simulink model "VECTOR_CONTROL_FOC_OF_IM_2023"  (R2023b)
settings: Solver=FixedStepDiscrete  StartTime=0.0  StopTime=1  RelTol=1e-3
PreLoadFcn:
  | Ts=2e-6;
InitFcn:
  | clc;
  | clear all;
  | % All Parameters
  | Ts=2e-6; %Sampling time
  | S=50*746; %nominal power
  | Vs=460; %Stator voltage
  | f=50; %Supply frequency
  | Rs=0.087; %Stator resistance
  | Rr=0.228; %Rotor resistance
  | Lls=0.0001; %Stator inductance
  | Llr=0.0008; %Rotor inductance
  | Lm=0.0347;
  | P=4; %Number of Poles
  | Tr=(Llr+Lm)/Rr; %Time constant
  | J=0.662; %Inertia
  | F=0.1; %Friction factor
  | Ls=Lls+Lm;
  | Lr=Llr+Lm;
undefined symbols (not defined in the file): DiscIntNeverNeededParam
libraries: slpidlib x3, spsVoltageMeasurementLib x3, spsAsynchronousMachineSIUnitsLib x1, spsSawtoothGeneratorLib x1, simulink_extras x1, spsUniversalBridgeLib x1, spsDCVoltageSourceLib x1, sps_lib x1, spsStairGeneratorLib x1
settings Model: Creator=ShahRukh
settings SolverCC: AlgebraicLoopSolver=TrustRegion
settings DataIOCC: ReturnWorkspaceOutputs=off
settings DebuggingCC: UnconnectedInputMsg=warning  UnconnectedOutputMsg=warning  UnconnectedLineMsg=warning  ArithmeticOperatorsInVariantConditions=warning
settings ModelReferenceCC: EnableRefExpFcnMdlSchedulingChecks=on
settings SFSimCC: SimUseLocalCustomCode=off  CustomCodeUndefinedFunction=UseInterfaceOnly
settings RTWCC: RTWUseLocalCustomCode=off
settings ConfigComp: CovBoundaryAbsTol=1.0e-5
settings SimscapeCC: SimscapeLogDataHistory=10000

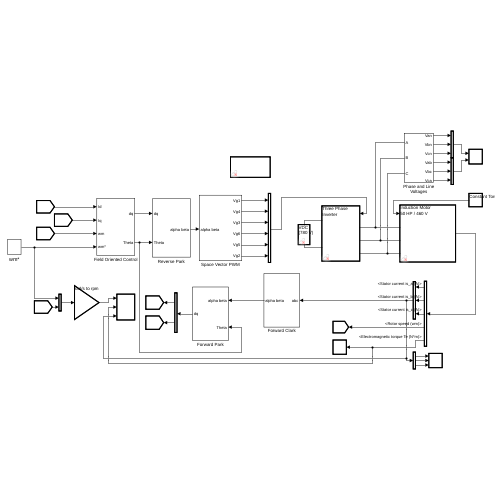
[thumbnail: Simulink's stored preview of the top-level diagram]
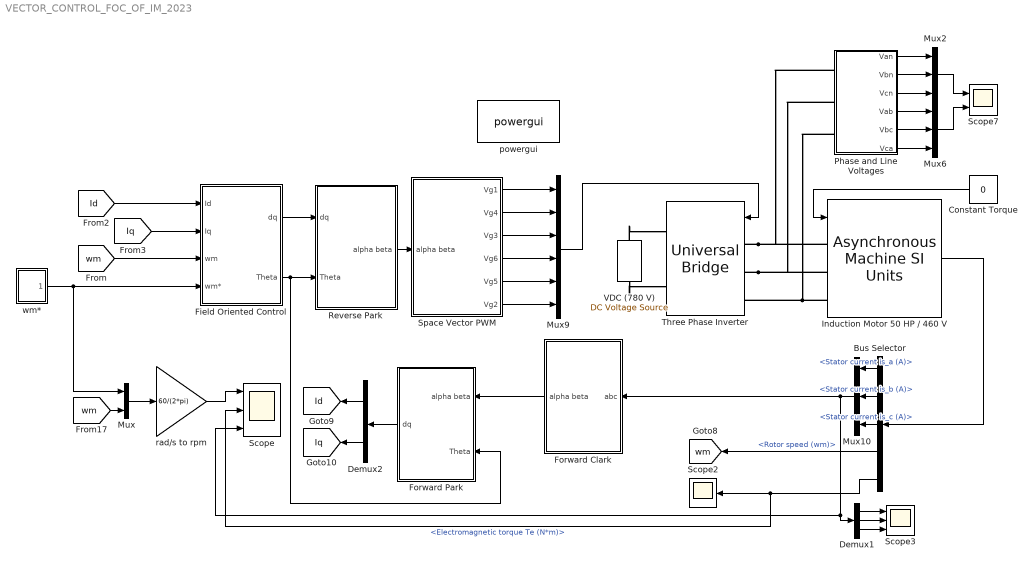
== system VECTOR_CONTROL_FOC_OF_IM_2023 ==
  Bus Selector : BusSelector  OutputSignals=Stator measurements.Stator current is_a (A),Stator measurements.Stator current is_b (A),Stator measurements.Stator current is_c (A),Mechanical.Rotor speed (wm),Mechanical.Electromagnetic torque Te (N*m)
  Constant Torque : Constant  Value=0
  Demux1 : Demux  Outputs=3
  Demux2 : Demux  Outputs=2
  Field Oriented Control : Subsystem
  Forward Clark : Subsystem
  Forward Park : Subsystem
  Induction Motor 50 HP / 460 V : spsAsynchronousMachineSIUnitsLib/Asynchronous Machine SI Units  RotorType=Squirrel-cage  PresetModel=No  MechanicalLoad=Torque Tm  ShowDetailedParameters=on  ReferenceFrame=Stationary  Units=SI  MeasurementBus=off  NominalParameters=[ S, Vs, f ]  VoltageRatio=1  Stator=[ Rs Lls ]  Rotor="[ Rr  Llr ]"  Cage1=[ 0.022 0.226/377]  Cage2=[ 0.022 0.226/377]  Lm=Lm  Mechanical="[J  F P/2 ]"  PolePairs=2  InitialConditions="[ 1, 0 ,  0 , 0 , 0 , 0 , 0 , 0 ]"  SimulateSaturation=off  Saturation=[0 0;0 0]  LoadFlowParameters=0  TsPowergui=0  TsBlock=-1  IterativeModel=Trapezoidal non iterative  IterativeDiscreteModel=Trapezoidal non iterative  Pmec=0
      settings: AttributesFormatString=\n
  Mux : Mux  Inputs=2
  Mux10 : Mux  Inputs=3
  Mux2 : Mux  Inputs=3
  Mux6 : Mux  Inputs=3
  Mux9 : Mux  Inputs=6
  Phase and Line Voltages : Subsystem
  Reverse Park : Subsystem
  Scope : Scope  NumInputPorts=3
  Scope2 : Scope
  Scope3 : Scope  NumInputPorts=3
  Scope7 : Scope  NumInputPorts=2
  Space Vector PWM : Subsystem
  Three Phase Inverter : spsUniversalBridgeLib/Universal Bridge  Arms=3  SnubberResistance=1000  SnubberCapacitance=inf  Device=IGBT / Diodes  Ron=1e-3  Lon=0  ForwardVoltages="[  0.8  0.8  ]"  ForwardVoltage=.8  GTOparameters=[ 1e-6 , 1e-6 ]  IGBTparameters=[ 1e-6 , 2e-6 ]  Measurements=None  Measurements_2=None  converterType=Rectifier
      settings: AttributesFormatString=\n
  VDC (780 V) : spsDCVoltageSourceLib/DC Voltage Source  Description=source block  Amplitude=780  Measurements=None
      settings: AttributesFormatString=\n
  powergui : sps_lib/powergui  Priority=2  SimulationMode=Discrete  SampleTime=Ts  frequency=60  Iterations=50  frequencyindice=0  Pbase=100e6  ErrMax=1e-4  UnitsV=kV  UnitsW=MW  buscounter=0  FunctionMessages=off  echomessages=off  EnableUseOfTLC=off  CurrentSourceSwitches=off  DisableSnubberDevices=off  DisableRonSwitches=off  DisableVfSwitches=off  DisplayEquations=off  AutomaticDiscreteSolvers=off  SolverType=Tustin  Interpol=off  ExternalGateDelay=off  methode=off  Ts=0  x0status=blocks  SPID=off  SwTol=0  HookPort=off  NonlinearTolerance=1e-4  nMaxIteration=100  ContinueOnMaxIteration=off  RestoreLinks=warning  ResistiveCurrentMeasurement=off  Frange=[0:2:500]  Ylog=off  Xlog=on  ShowGrid=off  save=off  variable=ZData  structure=0  ZoomFFT=on  StartTime=0.0  cycles=1  DisplayStyle=off  fundamental=60  FreqAxis=off  MaxFrequency=1000  frequencyindicesteady=1  RmsSteady=1  display=off
  rad/s to rpm : Gain  Gain=60/(2*pi)
  wm* : Subsystem
  tag scope: Id=global, Iq=global, wm=global
  wires:
  Bus Selector/4 -> [wm]  "<Rotor speed (wm)>"
  Mux10/1 -> Scope/3, Demux1/1, Forward Clark/1(abc)
  Demux2/1 -> [Id]
  Mux6/1 -> Scope7/2
  Space Vector PWM/6(Vg2) -> Mux9/6
  Constant Torque/1 -> Induction Motor 50 HP / 460 V/1
  Phase and Line Voltages/3(Vcn) -> Mux2/3
  Phase and Line Voltages/5(Vbc) -> Mux6/2
  Space Vector PWM/2(Vg4) -> Mux9/2
  Phase and Line Voltages/2(Vbn) -> Mux2/2
  Mux2/1 -> Scope7/1
  Space Vector PWM/5(Vg5) -> Mux9/5
  Phase and Line Voltages/1(Van) -> Mux2/1
  Phase and Line Voltages/6(Vca) -> Mux6/3
  Bus Selector/2 -> Mux10/2  "<Stator current is_b (A)>"
  Forward Park/1(dq) -> Demux2/1
  Demux2/2 -> [Iq]
  Bus Selector/5 -> Scope/2, Scope2/1  "<Electromagnetic torque Te (N*m)>"
  Mux9/1 -> Three Phase Inverter/1
  Bus Selector/1 -> Mux10/1  "<Stator current is_a (A)>"
  Forward Clark/1(alpha beta) -> Forward Park/1(alpha beta)
  Phase and Line Voltages/4(Vab) -> Mux6/1
  Mux/1 -> rad/s to rpm/1
  Space Vector PWM/3(Vg3) -> Mux9/3
  [wm] -> Mux/2
  Induction Motor 50 HP / 460 V/1 -> Bus Selector/1
  Space Vector PWM/1(Vg1) -> Mux9/1
  rad/s to rpm/1 -> Scope/1
  Space Vector PWM/4(Vg6) -> Mux9/4
  Reverse Park/1(alpha beta) -> Space Vector PWM/1(alpha beta)
  Field Oriented Control/1(dq) -> Reverse Park/1(dq)
  Bus Selector/3 -> Mux10/3  "<Stator current is_c (A)>"
  wm*/1(" ") -> Mux/1, Field Oriented Control/4(wm*)
  [wm] -> Field Oriented Control/3(wm)
  [Id] -> Field Oriented Control/1(Id)
  [Iq] -> Field Oriented Control/2(Iq)
  Field Oriented Control/2(Theta) -> Forward Park/2(Theta), Reverse Park/2(Theta)
  Demux1/1 -> Scope3/1
  Demux1/2 -> Scope3/2
  Demux1/3 -> Scope3/3
  connections:
  Three Phase Inverter/LConn1 -- Induction Motor 50 HP / 460 V/LConn1 -- Phase and Line Voltages/LConn1
  Induction Motor 50 HP / 460 V/LConn3 -- Three Phase Inverter/LConn3 -- Phase and Line Voltages/LConn3
  Three Phase Inverter/LConn2 -- Induction Motor 50 HP / 460 V/LConn2 -- Phase and Line Voltages/LConn2
  VDC (780 V)/RConn1 -- Three Phase Inverter/RConn1
  VDC (780 V)/LConn1 -- Three Phase Inverter/RConn2

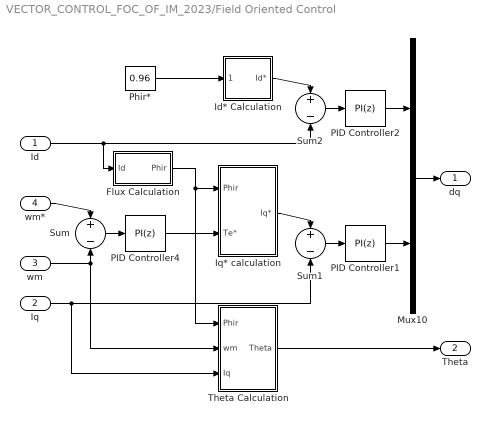
== system VECTOR_CONTROL_FOC_OF_IM_2023/Field Oriented Control ==
  Id : Inport
  Iq : Inport  Port=2
  wm : Inport  Port=3
  wm* : Inport  Port=4
  Flux Calculation : Subsystem  mask(Flux Calcultation){}
      mask init:
      | NF=0.44572610323020e-6;
      | DF=[1 -0.99998715486734];
  Id* Calculation : Subsystem
  Iq* calculation : Subsystem
  Mux10 : Mux  Inputs=2
  PID Controller1 : slpidlib/PID Controller  Controller=PI  Form=Parallel  TimeDomain=Discrete-time  UseExternalTs=off  SampleTime=-1  IntegratorMethod=Forward Euler  FilterMethod=Forward Euler  ControllerParametersSource=internal  P=100  I=26  UseKiTs=off  D=30  N=100  UseFilter=on  TunerSelectOption=Transfer Function Based (PID Tuner App)  InitialConditionSource=internal  InitialConditionForIntegrator=0  InitialConditionForFilter=0  DifferentiatorICPrevScaledInput=0  ExternalReset=none  TrackingMode=off  Kt=1  LimitOutput=off  SatLimitsSource=internal  UpperSaturationLimit=inf  LowerSaturationLimit=-inf  LinearizeAsGain=on  AntiWindupMode=none  Kb=1  LimitIntegrator=off  UpperIntegratorSaturationLimit=inf  LowerIntegratorSaturationLimit=-inf  POutMin=[]  POutMax=[]  IOutMin=[]  IOutMax=[]  DOutMin=[]  DOutMax=[]  NOutMin=[]  NOutMax=[]  SumOutMin=[]  SumOutMax=[]  SaturationOutMin=[]  SaturationOutMax=[]  PParamMin=[]  PParamMax=[]  IParamMin=[]  IParamMax=[]  DParamMin=[]  DParamMax=[]  NParamMin=[]  NParamMax=[]  KbParamMin=[]  KbParamMax=[]  KtParamMin=[]  KtParamMax=[]  KbOutMin=[]  KbOutMax=[]  KtOutMin=[]  KtOutMax=[]  IntegratorOutMin=[]  IntegratorOutMax=[]  FilterOutMin=[]  FilterOutMax=[]  SumI1OutMin=[]  SumI1OutMax=[]  SumI2OutMin=[]  SumI2OutMax=[]  SumI3OutMin=[]  SumI3OutMax=[]  SumI4OutMin=[]  SumI4OutMax=[]  SumDOutMin=[]  SumDOutMax=[]  DifferentiatorOutMin=[]  DifferentiatorOutMax=[]  FilterDiffOutCoefMin=[]  FilterDiffOutCoefMax=[]  ReciprocalOutMin=[]  ReciprocalOutMax=[]  SumDenOutMin=[]  SumDenOutMax=[]  SumNumOutMin=[]  SumNumOutMax=[]  DivideOutMin=[]  DivideOutMax=[]  UdiffTsProdOutMin=[]  UdiffTsProdOutMax=[]  NTsProdOutMin=[]  NTsProdOutMax=[]  UintegralTsProdOutMin=[]  UintegralTsProdOutMax=[]  UngainTsProdOutMin=[]  UngainTsProdOutMax=[]  ClampingZeroOutDataTypeStr=Inherit: Inherit via back propagation  ClampingZeroOutMin=[]  ClampingZeroOutMax=[]  FilterDenConstantOutDataTypeStr=Inherit: Inherit via back propagation  FilterDenConstantOutMin=[]  FilterDenConstantOutMax=[]  PCopyOutDataTypeStr=Inherit: Inherit via back propagation  PCopyOutMin=[]  PCopyOutMax=[]  NCopyOutDataTypeStr=Inherit: Inherit via back propagation  NCopyOutMin=[]  NCopyOutMax=[]  IntegratorContinuousStateAttributes=''  IntegratorStateMustResolveToSignalObject=off  IntegratorRTWStateStorageClass=Auto  FilterContinuousStateAttributes=''  FilterStateMustResolveToSignalObject=off  FilterRTWStateStorageClass=Auto  ParallelPVariant=InternalParameters  IdealPVariant=Disabled  IVariant=InternalParameters  DVariant=Disabled  IntegratorVariant=Discrete  SatVariant=Disabled  AWVariant=Passthrough  PCopyVariant=Disabled  TRVariant=Disabled  FdbkBlocksVariant=Forward  IdealPFdbkVariant=Disabled  SatFdbkVariant=Disabled  DerivativeFilterVariant=Disabled  NVariant=Disabled  NCopyVariant=Disabled_SignalSpec  FilterICVariant=Disabled  IntegratorICVariant=InternalICs  ExternalResetVariant=Disabled  TRSumVariant=Passthrough  SumFdbkVariant=Disabled  SumVariant=Sum_PI  TsampFilterVariant=InternalTs  TsampNgainVariant=Passthrough  TsampIntegralVariant=Disabled_SignalSpec  ExternalSaturationOutDataTypeStr=Inherit: Same as second input
  PID Controller2 : slpidlib/PID Controller  Controller=PI  Form=Parallel  TimeDomain=Discrete-time  UseExternalTs=off  SampleTime=-1  IntegratorMethod=Forward Euler  FilterMethod=Forward Euler  ControllerParametersSource=internal  P=100  I=26  UseKiTs=off  D=30  N=100  UseFilter=on  TunerSelectOption=Transfer Function Based (PID Tuner App)  InitialConditionSource=internal  InitialConditionForIntegrator=0  InitialConditionForFilter=0  DifferentiatorICPrevScaledInput=0  ExternalReset=none  TrackingMode=off  Kt=1  LimitOutput=off  SatLimitsSource=internal  UpperSaturationLimit=inf  LowerSaturationLimit=-inf  LinearizeAsGain=on  AntiWindupMode=none  Kb=1  LimitIntegrator=off  UpperIntegratorSaturationLimit=inf  LowerIntegratorSaturationLimit=-inf  POutMin=[]  POutMax=[]  IOutMin=[]  IOutMax=[]  DOutMin=[]  DOutMax=[]  NOutMin=[]  NOutMax=[]  SumOutMin=[]  SumOutMax=[]  SaturationOutMin=[]  SaturationOutMax=[]  PParamMin=[]  PParamMax=[]  IParamMin=[]  IParamMax=[]  DParamMin=[]  DParamMax=[]  NParamMin=[]  NParamMax=[]  KbParamMin=[]  KbParamMax=[]  KtParamMin=[]  KtParamMax=[]  KbOutMin=[]  KbOutMax=[]  KtOutMin=[]  KtOutMax=[]  IntegratorOutMin=[]  IntegratorOutMax=[]  FilterOutMin=[]  FilterOutMax=[]  SumI1OutMin=[]  SumI1OutMax=[]  SumI2OutMin=[]  SumI2OutMax=[]  SumI3OutMin=[]  SumI3OutMax=[]  SumI4OutMin=[]  SumI4OutMax=[]  SumDOutMin=[]  SumDOutMax=[]  DifferentiatorOutMin=[]  DifferentiatorOutMax=[]  FilterDiffOutCoefMin=[]  FilterDiffOutCoefMax=[]  ReciprocalOutMin=[]  ReciprocalOutMax=[]  SumDenOutMin=[]  SumDenOutMax=[]  SumNumOutMin=[]  SumNumOutMax=[]  DivideOutMin=[]  DivideOutMax=[]  UdiffTsProdOutMin=[]  UdiffTsProdOutMax=[]  NTsProdOutMin=[]  NTsProdOutMax=[]  UintegralTsProdOutMin=[]  UintegralTsProdOutMax=[]  UngainTsProdOutMin=[]  UngainTsProdOutMax=[]  ClampingZeroOutDataTypeStr=Inherit: Inherit via back propagation  ClampingZeroOutMin=[]  ClampingZeroOutMax=[]  FilterDenConstantOutDataTypeStr=Inherit: Inherit via back propagation  FilterDenConstantOutMin=[]  FilterDenConstantOutMax=[]  PCopyOutDataTypeStr=Inherit: Inherit via back propagation  PCopyOutMin=[]  PCopyOutMax=[]  NCopyOutDataTypeStr=Inherit: Inherit via back propagation  NCopyOutMin=[]  NCopyOutMax=[]  IntegratorContinuousStateAttributes=''  IntegratorStateMustResolveToSignalObject=off  IntegratorRTWStateStorageClass=Auto  FilterContinuousStateAttributes=''  FilterStateMustResolveToSignalObject=off  FilterRTWStateStorageClass=Auto  ParallelPVariant=InternalParameters  IdealPVariant=Disabled  IVariant=InternalParameters  DVariant=Disabled  IntegratorVariant=Discrete  SatVariant=Disabled  AWVariant=Passthrough  PCopyVariant=Disabled  TRVariant=Disabled  FdbkBlocksVariant=Forward  IdealPFdbkVariant=Disabled  SatFdbkVariant=Disabled  DerivativeFilterVariant=Disabled  NVariant=Disabled  NCopyVariant=Disabled_SignalSpec  FilterICVariant=Disabled  IntegratorICVariant=InternalICs  ExternalResetVariant=Disabled  TRSumVariant=Passthrough  SumFdbkVariant=Disabled  SumVariant=Sum_PI  TsampFilterVariant=InternalTs  TsampNgainVariant=Passthrough  TsampIntegralVariant=Disabled_SignalSpec  ExternalSaturationOutDataTypeStr=Inherit: Same as second input
  PID Controller4 : slpidlib/PID Controller  Controller=PI  Form=Parallel  TimeDomain=Discrete-time  UseExternalTs=off  SampleTime=-1  IntegratorMethod=Forward Euler  FilterMethod=Forward Euler  ControllerParametersSource=internal  P=20  I=26  UseKiTs=off  D=0  N=100  UseFilter=on  TunerSelectOption=Transfer Function Based (PID Tuner App)  InitialConditionSource=internal  InitialConditionForIntegrator=0  InitialConditionForFilter=0  DifferentiatorICPrevScaledInput=0  ExternalReset=none  TrackingMode=off  Kt=1  LimitOutput=off  SatLimitsSource=internal  UpperSaturationLimit=600  LowerSaturationLimit=-600  LinearizeAsGain=on  AntiWindupMode=none  Kb=1  LimitIntegrator=off  UpperIntegratorSaturationLimit=inf  LowerIntegratorSaturationLimit=-inf  POutMin=[]  POutMax=[]  IOutMin=[]  IOutMax=[]  DOutMin=[]  DOutMax=[]  NOutMin=[]  NOutMax=[]  SumOutMin=[]  SumOutMax=[]  SaturationOutMin=[]  SaturationOutMax=[]  PParamMin=[]  PParamMax=[]  IParamMin=[]  IParamMax=[]  DParamMin=[]  DParamMax=[]  NParamMin=[]  NParamMax=[]  KbParamMin=[]  KbParamMax=[]  KtParamMin=[]  KtParamMax=[]  KbOutMin=[]  KbOutMax=[]  KtOutMin=[]  KtOutMax=[]  IntegratorOutMin=[]  IntegratorOutMax=[]  FilterOutMin=[]  FilterOutMax=[]  SumI1OutMin=[]  SumI1OutMax=[]  SumI2OutMin=[]  SumI2OutMax=[]  SumI3OutMin=[]  SumI3OutMax=[]  SumI4OutMin=[]  SumI4OutMax=[]  SumDOutMin=[]  SumDOutMax=[]  DifferentiatorOutMin=[]  DifferentiatorOutMax=[]  FilterDiffOutCoefMin=[]  FilterDiffOutCoefMax=[]  ReciprocalOutMin=[]  ReciprocalOutMax=[]  SumDenOutMin=[]  SumDenOutMax=[]  SumNumOutMin=[]  SumNumOutMax=[]  DivideOutMin=[]  DivideOutMax=[]  UdiffTsProdOutMin=[]  UdiffTsProdOutMax=[]  NTsProdOutMin=[]  NTsProdOutMax=[]  UintegralTsProdOutMin=[]  UintegralTsProdOutMax=[]  UngainTsProdOutMin=[]  UngainTsProdOutMax=[]  ClampingZeroOutDataTypeStr=Inherit: Inherit via back propagation  ClampingZeroOutMin=[]  ClampingZeroOutMax=[]  FilterDenConstantOutDataTypeStr=Inherit: Inherit via back propagation  FilterDenConstantOutMin=[]  FilterDenConstantOutMax=[]  PCopyOutDataTypeStr=Inherit: Inherit via back propagation  PCopyOutMin=[]  PCopyOutMax=[]  NCopyOutDataTypeStr=Inherit: Inherit via back propagation  NCopyOutMin=[]  NCopyOutMax=[]  IntegratorContinuousStateAttributes=''  IntegratorStateMustResolveToSignalObject=off  IntegratorRTWStateStorageClass=Auto  FilterContinuousStateAttributes=''  FilterStateMustResolveToSignalObject=off  FilterRTWStateStorageClass=Auto  ParallelPVariant=InternalParameters  IdealPVariant=Disabled  IVariant=InternalParameters  DVariant=Disabled  IntegratorVariant=Discrete  SatVariant=Disabled  AWVariant=Passthrough  PCopyVariant=Disabled  TRVariant=Disabled  FdbkBlocksVariant=Forward  IdealPFdbkVariant=Disabled  SatFdbkVariant=Disabled  DerivativeFilterVariant=Disabled  NVariant=Disabled  NCopyVariant=Disabled_SignalSpec  FilterICVariant=Disabled  IntegratorICVariant=InternalICs  ExternalResetVariant=Disabled  TRSumVariant=Passthrough  SumFdbkVariant=Disabled  SumVariant=Sum_PI  TsampFilterVariant=InternalTs  TsampNgainVariant=Passthrough  TsampIntegralVariant=Disabled_SignalSpec  ExternalSaturationOutDataTypeStr=Inherit: Same as second input
  Phir* : Constant  Value=0.96
  Sum : Sum  Inputs=+-
  Sum1 : Sum  Inputs=+-
  Sum2 : Sum  Inputs=+-
  Theta Calculation : Subsystem
  dq : Outport  VectorParamsAs1DForOutWhenUnconnected=off
  Theta : Outport  Port=2  VectorParamsAs1DForOutWhenUnconnected=off
  wires:
  wm*/1 -> Sum/1
  Phir*/1 -> Id* Calculation/1(Phir*)
  Iq* calculation/1(Iq*) -> Sum1/1
  wm/1 -> Theta Calculation/2(wm), Sum/2
  Theta Calculation/1(Theta) -> Theta/1
  Id/1 -> Flux Calculation/1(Id), Sum2/2
  Mux10/1 -> dq/1
  Id* Calculation/1(Id*) -> Sum2/1
  PID Controller4/1 -> Iq* calculation/2(Te*)
  Sum1/1 -> PID Controller1/1
  Iq/1 -> Sum1/2, Theta Calculation/3(Iq)
  PID Controller2/1 -> Mux10/1
  PID Controller1/1 -> Mux10/2
  Sum2/1 -> PID Controller2/1
  Sum/1 -> PID Controller4/1
  Flux Calculation/1(Phir) -> Theta Calculation/1(Phir), Iq* calculation/1(Phir)

== system VECTOR_CONTROL_FOC_OF_IM_2023/Forward Clark ==
  abc : Inport
  Mux5 : Mux  Inputs=2
  alpha : Fcn  Expr=((2/3)*u(1))-((1/3)*u(2))-((1/3)*u(3))
  beta : Fcn  Expr=((0)*u(1))+((1/sqrt(3))*u(2))-((1/sqrt(3))*u(3))
  alpha beta : Outport  VectorParamsAs1DForOutWhenUnconnected=off
  wires:
  Mux5/1 -> alpha beta/1
  alpha/1 -> Mux5/1
  beta/1 -> Mux5/2
  abc/1 -> beta/1, alpha/1

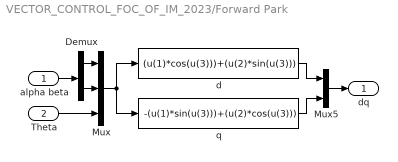
== system VECTOR_CONTROL_FOC_OF_IM_2023/Forward Park ==
  alpha beta : Inport
  Theta : Inport  Port=2
  Demux : Demux  Outputs=2
  Mux : Mux  Inputs=3
  Mux5 : Mux  Inputs=2
  d : Fcn  Expr=(u(1)*cos(u(3)))+(u(2)*sin(u(3)))
  q : Fcn  Expr=-(u(1)*sin(u(3)))+(u(2)*cos(u(3)))
  dq : Outport  VectorParamsAs1DForOutWhenUnconnected=off
  wires:
  Mux5/1 -> dq/1
  d/1 -> Mux5/1
  q/1 -> Mux5/2
  Mux/1 -> q/1, d/1
  alpha beta/1 -> Demux/1
  Demux/1 -> Mux/1
  Demux/2 -> Mux/2
  Theta/1 -> Mux/3

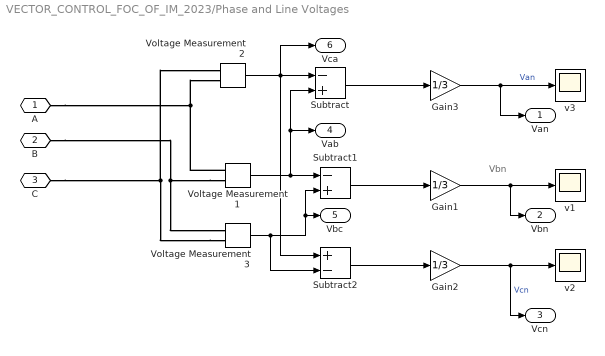
== system VECTOR_CONTROL_FOC_OF_IM_2023/Phase and Line Voltages ==
  note: Vbn
  Gain1 : Gain  Gain=1/3
  Gain2 : Gain  Gain=1/3
  Gain3 : Gain  Gain=1/3
  Subtract : Sum  Inputs=-+
  Subtract1 : Sum  Inputs=-+
  Subtract2 : Sum  Inputs=+-
  Voltage Measurement1 : spsVoltageMeasurementLib/Voltage Measurement  PhasorSimulation=off  OutputType=Complex  PSBequivalent=0
  Voltage Measurement2 : spsVoltageMeasurementLib/Voltage Measurement  PhasorSimulation=off  OutputType=Complex  PSBequivalent=0
  Voltage Measurement3 : spsVoltageMeasurementLib/Voltage Measurement  PhasorSimulation=off  OutputType=Complex  PSBequivalent=0
  v1 : Scope
  v2 : Scope
  v3 : Scope
  A : PMIOPort  Side=Left
  B : PMIOPort  Port=2  Side=Left
  C : PMIOPort  Port=3  Side=Left
  Van : Outport  VectorParamsAs1DForOutWhenUnconnected=off
  Vbn : Outport  Port=2  VectorParamsAs1DForOutWhenUnconnected=off
  Vcn : Outport  Port=3  VectorParamsAs1DForOutWhenUnconnected=off
  Vab : Outport  Port=4  VectorParamsAs1DForOutWhenUnconnected=off
  Vbc : Outport  Port=5  VectorParamsAs1DForOutWhenUnconnected=off
  Vca : Outport  Port=6  VectorParamsAs1DForOutWhenUnconnected=off
  wires:
  Gain2/1 -> v2/1, Vcn/1  "Vcn"
  Subtract2/1 -> Gain2/1
  Gain1/1 -> v1/1, Vbn/1
  Subtract1/1 -> Gain1/1
  Voltage Measurement3/1 -> Subtract1/2, Vbc/1, Subtract2/2
  Gain3/1 -> v3/1, Van/1  "Van"
  Subtract/1 -> Gain3/1
  Voltage Measurement1/1 -> Vab/1, Subtract/2, Subtract1/1
  Voltage Measurement2/1 -> Vca/1, Subtract2/1, Subtract/1
  connections:
  Voltage Measurement1/LConn1 -- A/RConn1 -- Voltage Measurement2/LConn2
  Voltage Measurement1/LConn2 -- B/RConn1 -- Voltage Measurement3/LConn1
  Voltage Measurement3/LConn2 -- Voltage Measurement2/LConn1 -- C/RConn1

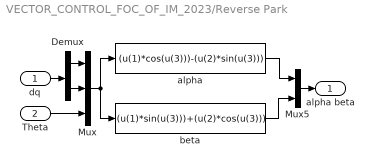
== system VECTOR_CONTROL_FOC_OF_IM_2023/Reverse Park ==
  dq : Inport
  Theta : Inport  Port=2
  Demux : Demux  Outputs=2
  Mux : Mux  Inputs=3
  Mux5 : Mux  Inputs=2
  alpha : Fcn  Expr=(u(1)*cos(u(3)))-(u(2)*sin(u(3)))
  beta : Fcn  Expr=(u(1)*sin(u(3)))+(u(2)*cos(u(3)))
  alpha beta : Outport  VectorParamsAs1DForOutWhenUnconnected=off
  wires:
  Mux5/1 -> alpha beta/1
  alpha/1 -> Mux5/1
  beta/1 -> Mux5/2
  Mux/1 -> beta/1, alpha/1
  dq/1 -> Demux/1
  Demux/1 -> Mux/1
  Demux/2 -> Mux/2
  Theta/1 -> Mux/3

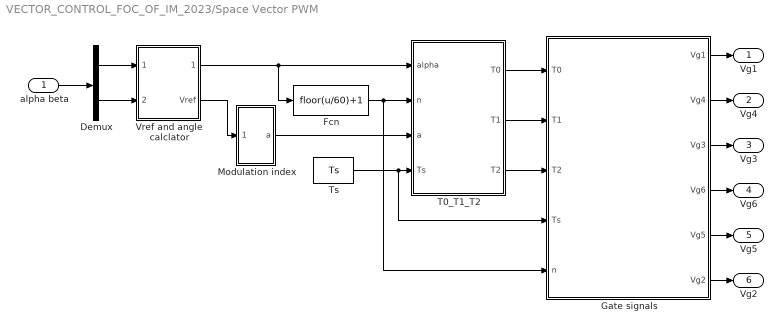
== system VECTOR_CONTROL_FOC_OF_IM_2023/Space Vector PWM ==
  alpha beta : Inport
  Demux : Demux  Outputs=2
  Fcn : Fcn  Expr=floor(u/60)+1
  Gate signals : Subsystem
  Modulation index : Subsystem
  T0_T1_T2 : Subsystem
  Ts : Constant  Value=Ts
  Vref and angle calclator : Subsystem
  Vg1 : Outport  VectorParamsAs1DForOutWhenUnconnected=off
  Vg4 : Outport  Port=2  VectorParamsAs1DForOutWhenUnconnected=off
  Vg3 : Outport  Port=3  VectorParamsAs1DForOutWhenUnconnected=off
  Vg6 : Outport  Port=4  VectorParamsAs1DForOutWhenUnconnected=off
  Vg5 : Outport  Port=5  VectorParamsAs1DForOutWhenUnconnected=off
  Vg2 : Outport  Port=6  VectorParamsAs1DForOutWhenUnconnected=off
  wires:
  Fcn/1 -> T0_T1_T2/2(n), Gate signals/5(n)
  T0_T1_T2/3(T2) -> Gate signals/3(T2)
  Demux/2 -> Vref and angle calclator/2(Vbeta)
  Gate signals/5(Vg5) -> Vg5/1
  Gate signals/4(Vg6) -> Vg6/1
  Gate signals/2(Vg4) -> Vg4/1
  Gate signals/3(Vg3) -> Vg3/1
  Gate signals/1(Vg1) -> Vg1/1
  Ts/1 -> Gate signals/4(Ts), T0_T1_T2/4(Ts)
  Gate signals/6(Vg2) -> Vg2/1
  T0_T1_T2/1(T0) -> Gate signals/1(T0)
  T0_T1_T2/2(T1) -> Gate signals/2(T1)
  Vref and angle calclator/2(Vref) -> Modulation index/1(Vref)
  Modulation index/1(a) -> T0_T1_T2/3(a)
  Vref and angle calclator/1(alpha) -> Fcn/1, T0_T1_T2/1(alpha)
  alpha beta/1 -> Demux/1
  Demux/1 -> Vref and angle calclator/1(Valpha)

== system VECTOR_CONTROL_FOC_OF_IM_2023/wm* ==
  Stair Generator : spsStairGeneratorLib/Stair Generator  t=[0 1 2 3 4 5 6 7 8 9]  e=[50 95 60 105 70 95 90 95 80 55]  Ts=Ts
  " " : Outport  VectorParamsAs1DForOutWhenUnconnected=off
  wires:
  Stair Generator/1 -> " "/1

== system VECTOR_CONTROL_FOC_OF_IM_2023/Field Oriented Control/Flux Calculation ==
  Id : Inport
  First Order Low Pass Filter : DiscreteTransferFcn  Numerator=[Lm*Ts/Tr]  Denominator=[1 (Ts-Tr)/Tr]
  Phir : Outport  VectorParamsAs1DForOutWhenUnconnected=off
  wires:
  Id/1 -> First Order Low Pass Filter/1
  First Order Low Pass Filter/1 -> Phir/1

== system VECTOR_CONTROL_FOC_OF_IM_2023/Field Oriented Control/Id* Calculation ==
  Phir* : Inport
  Gain : Gain  Gain=1/Lm  SaturateOnIntegerOverflow=on  OutDataTypeStr=Inherit: Same as input  ParamDataTypeStr=Inherit: Same as input
  Id* : Outport  VectorParamsAs1DForOutWhenUnconnected=off
  wires:
  Gain/1 -> Id*/1
  Phir*/1 -> Gain/1

== system VECTOR_CONTROL_FOC_OF_IM_2023/Field Oriented Control/Iq* calculation ==
  Phir : Inport
  Te* : Inport  Port=2
  Fcn : Fcn  Expr=(2/3)*(2/P)*((Llr+Lm)/Lm)*(u(1)/(u(2)+1e-3))
  Mux : Mux  Inputs=2
  Iq* : Outport  InitialOutput=0  VectorParamsAs1DForOutWhenUnconnected=off
  wires:
  Phir/1 -> Mux/2
  Fcn/1 -> Iq*/1
  Te*/1 -> Mux/1
  Mux/1 -> Fcn/1

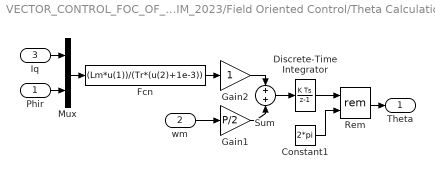
== system VECTOR_CONTROL_FOC_OF_IM_2023/Field Oriented Control/Theta Calculation ==
  Phir : Inport
  wm : Inport  Port=2
  Iq : Inport  Port=3
  Constant1 : Constant  Value=2*pi
  Discrete-Time Integrator : DiscreteIntegrator  SampleTime=Ts  ICPrevOutput=DiscIntNeverNeededParam  ICPrevScaledInput=DiscIntNeverNeededParam
  Fcn : Fcn  Expr=(Lm*u(1))/(Tr*(u(2)+1e-3))
  Gain1 : Gain  Gain=P/2  SaturateOnIntegerOverflow=on  OutDataTypeStr=Inherit: Same as input  ParamDataTypeStr=Inherit: Same as input
  Gain2 : Gain  SaturateOnIntegerOverflow=on  OutDataTypeStr=Inherit: Same as input  ParamDataTypeStr=Inherit: Same as input
  Mux : Mux  Inputs=2
  Rem : Math  Operator=rem  SignedPower=on
  Sum : Sum
  Theta : Outport  InitialOutput=0  VectorParamsAs1DForOutWhenUnconnected=off
  wires:
  Sum/1 -> Discrete-Time Integrator/1
  Gain1/1 -> Sum/2
  Gain2/1 -> Sum/1
  wm/1 -> Gain1/1
  Fcn/1 -> Gain2/1
  Phir/1 -> Mux/2
  Iq/1 -> Mux/1
  Mux/1 -> Fcn/1
  Constant1/1 -> Rem/2
  Discrete-Time Integrator/1 -> Rem/1
  Rem/1 -> Theta/1

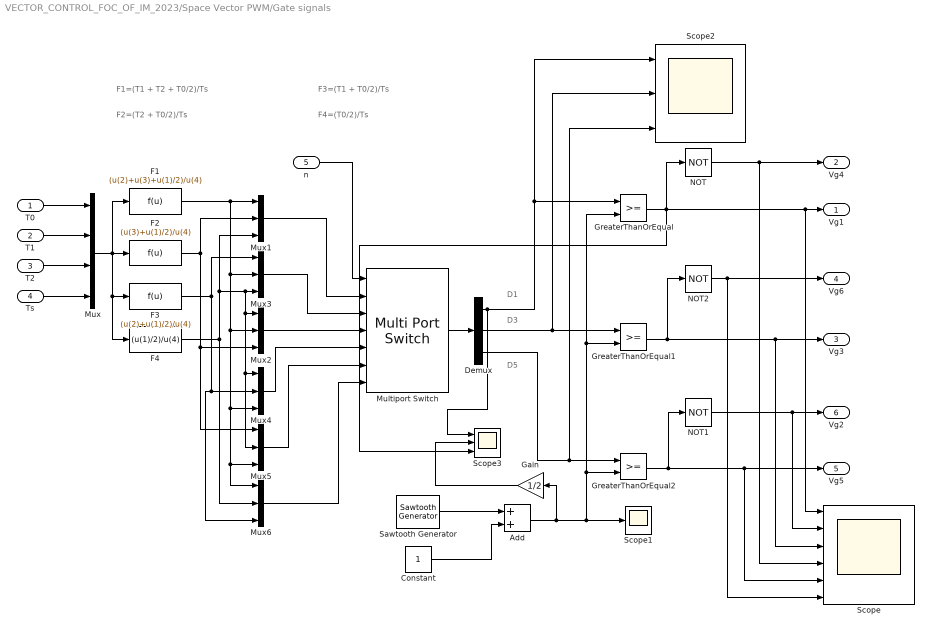
== system VECTOR_CONTROL_FOC_OF_IM_2023/Space Vector PWM/Gate signals ==
  note: D1
  note: F1=(T1 + T2 + T0/2)/Ts
  note: F2=(T2 + T0/2)/Ts
  note: F3=(T1 + T0/2)/Ts
  note: F4=(T0/2)/Ts
  note: D3
  note: D5
  T0 : Inport
  T1 : Inport  Port=2
  T2 : Inport  Port=3
  Ts : Inport  Port=4
  n : Inport  Port=5
  Add : Sum
  Constant : Constant
  Demux : Demux  Outputs=3
  F1 : Fcn  Expr=(u(2)+u(3)+u(1)/2)/u(4)
  F2 : Fcn  Expr=(u(3)+u(1)/2)/u(4)
  F3 : Fcn  Expr=(u(2)+u(1)/2)/u(4)
  F4 : Fcn  Expr=(u(1)/2)/u(4)
  Gain : Gain  Gain=1/2
  GreaterThanOrEqual : RelationalOperator  OutDataTypeStr=boolean  RndMeth=Simplest  InputSameDT=off
  GreaterThanOrEqual1 : RelationalOperator  OutDataTypeStr=boolean  RndMeth=Simplest  InputSameDT=off
  GreaterThanOrEqual2 : RelationalOperator  OutDataTypeStr=boolean  RndMeth=Simplest  InputSameDT=off
  Multiport Switch : MultiPortSwitch  Inputs=6  DiagnosticForDefault=None  SaturateOnIntegerOverflow=off  InputSameDT=off
  Mux : Mux
  Mux{1..6} (6 alike) : Mux  Inputs=3
  NOT : Logic  Operator=NOT  IconShape=distinctive  AllPortsSameDT=off  OutDataTypeStr=boolean
  NOT1 : Logic  Operator=NOT  IconShape=distinctive  AllPortsSameDT=off  OutDataTypeStr=boolean
  NOT2 : Logic  Operator=NOT  IconShape=distinctive  AllPortsSameDT=off  OutDataTypeStr=boolean
  Sawtooth Generator : spsSawtoothGeneratorLib/Sawtooth Generator  Freq=5e3  Phase=0  Ts=0
  Scope : Scope  NumInputPorts=6
  Scope1 : Scope
  Scope2 : Scope  NumInputPorts=3
  Scope3 : Scope  NumInputPorts=3
  Vg1 : Outport  VectorParamsAs1DForOutWhenUnconnected=off
  Vg4 : Outport  Port=2  VectorParamsAs1DForOutWhenUnconnected=off
  Vg3 : Outport  Port=3  VectorParamsAs1DForOutWhenUnconnected=off
  Vg6 : Outport  Port=4  VectorParamsAs1DForOutWhenUnconnected=off
  Vg5 : Outport  Port=5  VectorParamsAs1DForOutWhenUnconnected=off
  Vg2 : Outport  Port=6  VectorParamsAs1DForOutWhenUnconnected=off
  wires:
  Demux/2 -> GreaterThanOrEqual1/1, Scope2/2
  Sawtooth Generator/1 -> Add/1
  GreaterThanOrEqual/1 -> Scope3/3, Scope/1, Vg1/1, NOT/1
  GreaterThanOrEqual1/1 -> NOT2/1, Scope/3, Vg3/1
  GreaterThanOrEqual2/1 -> NOT1/1, Scope/5, Vg5/1
  NOT/1 -> Scope/4, Vg4/1
  NOT1/1 -> Scope/2, Vg2/1
  NOT2/1 -> Scope/6, Vg6/1
  n/1 -> Multiport Switch/1
  T0/1 -> Mux/1
  T1/1 -> Mux/2
  T2/1 -> Mux/3
  Ts/1 -> Mux/4
  Mux/1 -> F1/1, F2/1, F4/1, F3/1
  Demux/3 -> GreaterThanOrEqual2/1, Scope2/3
  Add/1 -> Gain/1, Scope1/1, GreaterThanOrEqual2/2, GreaterThanOrEqual1/2, GreaterThanOrEqual/2
  Constant/1 -> Add/2
  Multiport Switch/1 -> Demux/1
  Demux/1 -> Scope3/1, GreaterThanOrEqual/1, Scope2/1
  Mux6/1 -> Multiport Switch/7
  Mux5/1 -> Multiport Switch/6
  Mux4/1 -> Multiport Switch/5
  Mux2/1 -> Multiport Switch/4
  Mux3/1 -> Multiport Switch/3
  Mux1/1 -> Multiport Switch/2
  F1/1 -> Mux6/1, Mux5/3, Mux4/3, Mux2/2, Mux3/2, Mux1/1
  F2/1 -> Mux1/2, Mux5/1, Mux2/3
  F4/1 -> Mux6/2, Mux5/2, Mux4/1, Mux2/1, Mux3/3, Mux1/3
  F3/1 -> Mux6/3, Mux4/2, Mux3/1
  Gain/1 -> Scope3/2

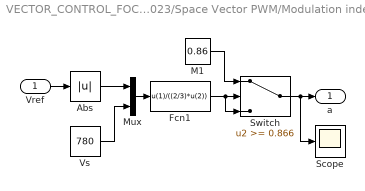
== system VECTOR_CONTROL_FOC_OF_IM_2023/Space Vector PWM/Modulation index ==
  Vref : Inport
  Abs : Abs  SaturateOnIntegerOverflow=off
  Fcn1 : Fcn  Expr=u(1)/((2/3)*u(2))
  M1 : Constant  Value=0.86
  Mux : Mux  Inputs=2
  Scope : Scope
  Switch : Switch  Threshold=0.866  SaturateOnIntegerOverflow=off  InputSameDT=off
  Vs : Constant  Value=780
  a : Outport  VectorParamsAs1DForOutWhenUnconnected=off
  wires:
  Fcn1/1 -> Switch/3, Switch/2
  Vs/1 -> Mux/2
  M1/1 -> Switch/1
  Vref/1 -> Abs/1
  Mux/1 -> Fcn1/1
  Switch/1 -> Scope/1, a/1
  Abs/1 -> Mux/1

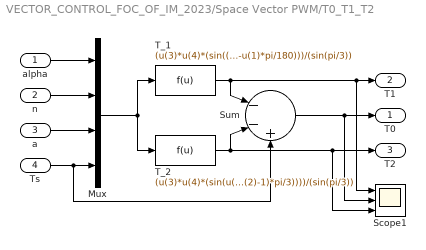
== system VECTOR_CONTROL_FOC_OF_IM_2023/Space Vector PWM/T0_T1_T2 ==
  alpha : Inport
  n : Inport  Port=2
  a : Inport  Port=3
  Ts : Inport  Port=4
  Mux : Mux
  Scope1 : Scope  NumInputPorts=3
  Sum : Sum  Inputs=|--+
  T_1 : Fcn  Expr=(u(3)*u(4)*(sin((u(2)*pi/3)-u(1)*pi/180)))/(sin(pi/3))
  T_2 : Fcn  Expr=(u(3)*u(4)*(sin(u(1)*pi/180-((u(2)-1)*pi/3))))/(sin(pi/3))
  T0 : Outport  VectorParamsAs1DForOutWhenUnconnected=off
  T1 : Outport  Port=2  VectorParamsAs1DForOutWhenUnconnected=off
  T2 : Outport  Port=3  VectorParamsAs1DForOutWhenUnconnected=off
  wires:
  Mux/1 -> T_2/1, T_1/1
  n/1 -> Mux/2
  a/1 -> Mux/3
  Ts/1 -> Sum/3, Mux/4
  T_2/1 -> Sum/2, Scope1/3, T2/1
  T_1/1 -> Scope1/1, T1/1, Sum/1
  Sum/1 -> Scope1/2, T0/1
  alpha/1 -> Mux/1

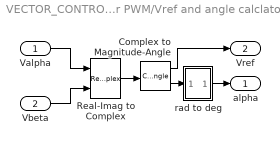
== system VECTOR_CONTROL_FOC_OF_IM_2023/Space Vector PWM/Vref and angle calclator ==
  Valpha : Inport
  Vbeta : Inport  Port=2
  Complex to Magnitude-Angle : ComplexToMagnitudeAngle
  Real-Imag to Complex : RealImagToComplex
  rad to deg : Subsystem
  alpha : Outport  VectorParamsAs1DForOutWhenUnconnected=off
  Vref : Outport  Port=2  VectorParamsAs1DForOutWhenUnconnected=off
  wires:
  Valpha/1 -> Real-Imag to Complex/1
  Real-Imag to Complex/1 -> Complex to Magnitude-Angle/1
  Vbeta/1 -> Real-Imag to Complex/2
  rad to deg/1(2D) -> alpha/1
  Complex to Magnitude-Angle/2 -> rad to deg/1(R)
  Complex to Magnitude-Angle/1 -> Vref/1

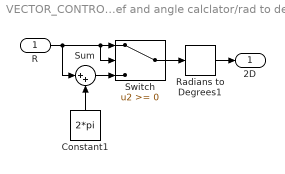
== system VECTOR_CONTROL_FOC_OF_IM_2023/Space Vector PWM/Vref and angle calclator/rad to deg ==
  R : Inport
  Constant1 : Constant  Value=2*pi
  Radians to Degrees1 : simulink_extras/Transformations/Radians to Degrees
  Sum : Sum  Inputs=|++
  Switch : Switch  SaturateOnIntegerOverflow=off  InputSameDT=off
  2D : Outport  VectorParamsAs1DForOutWhenUnconnected=off
  wires:
  R/1 -> Switch/2, Switch/1, Sum/1
  Radians to Degrees1/1 -> 2D/1
  Switch/1 -> Radians to Degrees1/1
  Sum/1 -> Switch/3
  Constant1/1 -> Sum/2
